simulink model "rx_20140505"  (R2012b)
settings: Solver=ode45  StartTime=0.0  StopTime=10000.0  RelTol=1e-3
libraries: xbsIndex_r4 x2064, casper_library_misc x67, xps_library x56, xbsReplacements_r4 x12, gavrt_library x3, casper_library_sources x2, simulink x1, casper_library_delays x1
(part 2 of 22)

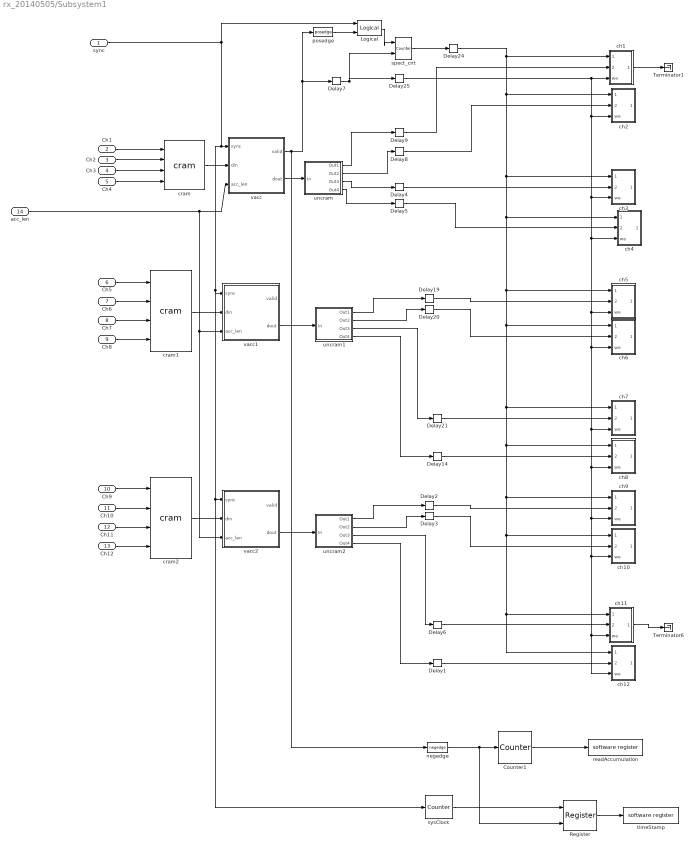
== system rx_20140505/Subsystem1 ==
  sync : Inport
  Ch1 : Inport  Port=2
  Ch2 : Inport  Port=3
  Ch3 : Inport  Port=4
  Ch4 : Inport  Port=5
  Ch5 : Inport  Port=6
  Ch6 : Inport  Port=7
  Ch7 : Inport  Port=8
  Ch8 : Inport  Port=9
  Ch9 : Inport  Port=10
  Ch10 : Inport  Port=11
  Ch11 : Inport  Port=12
  Ch12 : Inport  Port=13
  acc_len : Inport  Port=14
  Counter1 : xbsIndex_r4/Counter  cnt_type=Free Running  cnt_to=Inf  operation=Up  start_count=0  cnt_by_val=1  arith_type=Unsigned  n_bits=32  bin_pt=0  load_pin=off  rst=off  en=on  explicit_period=on  period=1  dbl_ovrd=off  use_behavioral_HDL=off  implementation=Fabric  block_type=counter
      settings: block_version=11.4
  Delay{1..6,8..9,14,19..21} (12 alike) : xbsIndex_r4/Delay  rst=off  infoeditControl=Selection of Reset will increase slice count due to use of real FFs and instead of SRLs  en=off  latency=2  dbl_ovrd=off  reg_retiming=on  block_type=delay
  Delay24 : xbsIndex_r4/Delay  rst=off  infoeditControl=Selection of Reset will increase slice count due to use of real FFs and instead of SRLs  en=off  latency=1  dbl_ovrd=off  reg_retiming=on  block_type=delay
  Delay25 : xbsIndex_r4/Delay  rst=off  infoeditControl=Selection of Reset will increase slice count due to use of real FFs and instead of SRLs  en=off  latency=1  dbl_ovrd=off  reg_retiming=on  block_type=delay
  Delay7 : xbsIndex_r4/Delay  rst=off  infoeditControl=Selection of Reset will increase slice count due to use of real FFs and instead of SRLs  en=off  latency=1  dbl_ovrd=off  reg_retiming=on  block_type=delay
  Logical : xbsIndex_r4/Logical  logical_function=OR  inputs=2  en=off  latency=0  precision=Full  arith_type=Unsigned  n_bits=16  bin_pt=0  align_bp=on  dbl_ovrd=off  block_type=logical
      settings: block_version=11.4
  Register : xbsIndex_r4/Register  init=0  rst=off  en=on  dbl_ovrd=off  block_type=register
      settings: block_version=11.4
  Terminator1 : Terminator
  Terminator6 : Terminator
  ch1 : Subsystem
  ch10 : Subsystem
  ch11 : Subsystem
  ch12 : Subsystem
  ch2 : Subsystem
  ch3 : Subsystem
  ch4 : Subsystem
  ch5 : Subsystem
  ch6 : Subsystem
  ch7 : Subsystem
  ch8 : Subsystem
  ch9 : Subsystem
  cram : gavrt_library/cram  num_slice=4
  cram1 : gavrt_library/cram  num_slice=4
  cram2 : gavrt_library/cram  num_slice=4
  negedge : casper_library_misc/negedge  Tag=Rising Edge Detector
  posedge : casper_library_misc/posedge  Tag=Rising Edge Detector
  readAccumulation : xps_library/software register  Tag=xps:sw_reg  io_dir=To Processor  arith_type=Unsigned  bitwidth=32  bin_pt=0  sample_period=1  gw_name=rx_20140505_Subsystem1_readAccumulation_user_data_in
  spect_cnt : xbsIndex_r4/Counter  cnt_type=Free Running  cnt_to=Inf  operation=Up  start_count=0  cnt_by_val=1  arith_type=Unsigned  n_bits=10  bin_pt=0  load_pin=off  rst=on  en=on  explicit_period=on  period=1  dbl_ovrd=off  use_behavioral_HDL=off  implementation=Fabric  use_rpm=off  block_type=counter
  sysClock : xbsIndex_r4/Counter  cnt_type=Free Running  cnt_to=Inf  operation=Up  start_count=0  cnt_by_val=1  arith_type=Unsigned  n_bits=32  bin_pt=0  load_pin=off  rst=on  en=off  explicit_period=on  period=1  dbl_ovrd=off  use_behavioral_HDL=off  implementation=Fabric  block_type=counter
      settings: block_version=11.4
  timeStamp : xps_library/software register  Tag=xps:sw_reg  io_dir=To Processor  arith_type=Unsigned  bitwidth=32  bin_pt=0  sample_period=1  gw_name=rx_20140505_Subsystem1_timeStamp_user_data_in
  uncram : Subsystem  AncestorBlock=gavrt_library/uncram  mask(uncram){num_slice=4, slice_width=64, bin_pt=0, arith_type=1}
      mask prompts: num_slice "Number of slices"; slice_width "Slice Width"; bin_pt "Output Binary Point"; arith_type "Output Arithmetic Type (0=Unsigned, 1=Signed)"
      mask help: Takes a concatenated input and slices it up into even pieces and reinterprets them as signed fixed point numbers with a given binary point.
      mask init:
      | uncram_init(gcb, ...
      |     'num_slice', num_slice, ...
      |     'slice_width', slice_width, ...
      |     'bin_pt', bin_pt, ...
      |     'arith_type', arith_type);
      settings: AttributesFormatString=Fix_64_0
  uncram1 : Subsystem  AncestorBlock=gavrt_library/uncram  mask(uncram){num_slice=4, slice_width=64, bin_pt=0, arith_type=1}
      mask prompts: num_slice "Number of slices"; slice_width "Slice Width"; bin_pt "Output Binary Point"; arith_type "Output Arithmetic Type (0=Unsigned, 1=Signed)"
      mask help: Takes a concatenated input and slices it up into even pieces and reinterprets them as signed fixed point numbers with a given binary point.
      mask init:
      | uncram_init(gcb, ...
      |     'num_slice', num_slice, ...
      |     'slice_width', slice_width, ...
      |     'bin_pt', bin_pt, ...
      |     'arith_type', arith_type);
      settings: AttributesFormatString=Fix_64_0
  uncram2 : Subsystem  AncestorBlock=gavrt_library/uncram  mask(uncram){num_slice=4, slice_width=64, bin_pt=0, arith_type=1}
      mask prompts: num_slice "Number of slices"; slice_width "Slice Width"; bin_pt "Output Binary Point"; arith_type "Output Arithmetic Type (0=Unsigned, 1=Signed)"
      mask help: Takes a concatenated input and slices it up into even pieces and reinterprets them as signed fixed point numbers with a given binary point.
      mask init:
      | uncram_init(gcb, ...
      |     'num_slice', num_slice, ...
      |     'slice_width', slice_width, ...
      |     'bin_pt', bin_pt, ...
      |     'arith_type', arith_type);
      settings: AttributesFormatString=Fix_64_0
  vacc : Subsystem  AncestorBlock=gavrt_library/vacc  mask(vacc){veclen=5, ninputs=4, max_accum=22, arith_type=1, in_bit_width=37, in_bin_pt=0, out_bit_width=64, out_bin_pt=0, register_din=0, add_latency=3, bram_latency=4, mux_latency=4}
      mask prompts: veclen "Vector Length (2^?)"; ninputs "Number of Simultaneous Vectors"; max_accum "Maximum # Accumulations (2^?)"; arith_type "Arithmetic Type (0=Unsigned, 1=Signed)"; in_bit_width "Input Bit Width"; in_bin_pt "Input Binary Point"; out_bit_width "Output Bit Width"; out_bin_pt "Output Binary Point"; register_din "Register Input Data  (1 = Enable Register Retiming on input delay)"; add_latency "Add Latency"; bram_latency "BRAM Latency"; mux_latency "Mux Latency"
      mask help:
      | Sync is expected the clock before the first data to be accumulated.
      | Use the Cram block to feed din for multiple simultaneous inputs.
      | acc_len is the number of vectors to sum.
      | valid is high while a valid accumulation is being clocked out on dout.
      | If only one sync pulse is provided, valid accumulations will repeatedly appear on dout as they become available.
      | Undesired behavior may occur if acc_len is changed without a new sync pulse.
      | Note: The output is an unsigned concatenation of the output streams. Thus, even with only one stream, the output must be recast before using.
      | Register Input Data controls the "Enable Register Retiming" parameter of the delays on 'din'.
      mask init:
      | vacc_init(gcb, ...
      |     'veclen', veclen, ...
      |     'ninputs', ninputs, ...
      |     'max_accum', max_accum, ...
      |     'arith_type', arith_type, ...
      |     'in_bit_width', in_bit_width, ...
      |     'in_bin_pt', in_bin_pt, ...
      |     'out_bit_width', out_bit_width, ...
      |     'out_bin_pt', out_bin_pt, ...
      |     'register_din', register_din, ...
      |     'add_latency', add_latency, ...
      |     'bram_latency', bram_latency, ...
      |     'mux_latency', mux_latency);
      settings: AttributesFormatString=|
      | vector length=32, inputs=4
      | max accumulations=2^22
  vacc1 : Subsystem  AncestorBlock=gavrt_library/vacc  mask(vacc){veclen=5, ninputs=4, max_accum=22, arith_type=1, in_bit_width=37, in_bin_pt=0, out_bit_width=64, out_bin_pt=0, register_din=0, add_latency=3, bram_latency=4, mux_latency=4}
      mask prompts: veclen "Vector Length (2^?)"; ninputs "Number of Simultaneous Vectors"; max_accum "Maximum # Accumulations (2^?)"; arith_type "Arithmetic Type (0=Unsigned, 1=Signed)"; in_bit_width "Input Bit Width"; in_bin_pt "Input Binary Point"; out_bit_width "Output Bit Width"; out_bin_pt "Output Binary Point"; register_din "Register Input Data  (1 = Enable Register Retiming on input delay)"; add_latency "Add Latency"; bram_latency "BRAM Latency"; mux_latency "Mux Latency"
      mask help:
      | Sync is expected the clock before the first data to be accumulated.
      | Use the Cram block to feed din for multiple simultaneous inputs.
      | acc_len is the number of vectors to sum.
      | valid is high while a valid accumulation is being clocked out on dout.
      | If only one sync pulse is provided, valid accumulations will repeatedly appear on dout as they become available.
      | Undesired behavior may occur if acc_len is changed without a new sync pulse.
      | Note: The output is an unsigned concatenation of the output streams. Thus, even with only one stream, the output must be recast before using.
      | Register Input Data controls the "Enable Register Retiming" parameter of the delays on 'din'.
      mask init: same as rx_20140505/Subsystem1/vacc
      settings: AttributesFormatString=|
      | vector length=32, inputs=4
      | max accumulations=2^22
  vacc2 : Subsystem  AncestorBlock=gavrt_library/vacc  mask(vacc){veclen=5, ninputs=4, max_accum=22, arith_type=1, in_bit_width=37, in_bin_pt=0, out_bit_width=64, out_bin_pt=0, register_din=0, add_latency=3, bram_latency=4, mux_latency=4}
      mask prompts: veclen "Vector Length (2^?)"; ninputs "Number of Simultaneous Vectors"; max_accum "Maximum # Accumulations (2^?)"; arith_type "Arithmetic Type (0=Unsigned, 1=Signed)"; in_bit_width "Input Bit Width"; in_bin_pt "Input Binary Point"; out_bit_width "Output Bit Width"; out_bin_pt "Output Binary Point"; register_din "Register Input Data  (1 = Enable Register Retiming on input delay)"; add_latency "Add Latency"; bram_latency "BRAM Latency"; mux_latency "Mux Latency"
      mask help:
      | Sync is expected the clock before the first data to be accumulated.
      | Use the Cram block to feed din for multiple simultaneous inputs.
      | acc_len is the number of vectors to sum.
      | valid is high while a valid accumulation is being clocked out on dout.
      | If only one sync pulse is provided, valid accumulations will repeatedly appear on dout as they become available.
      | Undesired behavior may occur if acc_len is changed without a new sync pulse.
      | Note: The output is an unsigned concatenation of the output streams. Thus, even with only one stream, the output must be recast before using.
      | Register Input Data controls the "Enable Register Retiming" parameter of the delays on 'din'.
      mask init: same as rx_20140505/Subsystem1/vacc
      settings: AttributesFormatString=|
      | vector length=32, inputs=4
      | max accumulations=2^22
  wires:
  ch1/1(Out1) -> Terminator1/1
  Delay4/1 -> ch3/2(data)
  uncram1/2(Out2) -> Delay20/1
  uncram1/3(Out3) -> Delay21/1
  Ch3/1 -> cram/3
  Ch4/1 -> cram/4
  Ch2/1 -> cram/2
  Ch1/1 -> cram/1
  cram/1 -> vacc/2(din)
  vacc/1(valid) -> posedge/1, Delay7/1, negedge/1
  Delay7/1 -> spect_cnt/2, Delay25/1
  vacc/2(dout) -> uncram/1(In)
  uncram/1(Out1) -> Delay9/1
  uncram/2(Out2) -> Delay8/1
  uncram/3(Out3) -> Delay4/1
  uncram/4(Out4) -> Delay5/1
  Delay8/1 -> ch2/2(data)
  Delay9/1 -> ch1/2(data)
  spect_cnt/1 -> Delay24/1
  Delay24/1 -> ch1/1(addr), ch2/1(addr), ch3/1(addr), ch4/1(addr), ch5/1(addr), ch6/1(addr), ch7/1(addr), ch8/1(addr), ch9/1(addr), ch10/1(addr), ch12/1(addr), ch11/1(addr)
  Delay25/1 -> ch1/3(we), ch2/3(we), ch3/3(we), ch4/3(we), ch5/3(we), ch6/3(we), ch7/3(we), ch8/3(we), ch9/3(we), ch10/3(we), ch12/3(we), ch11/3(we)
  Delay5/1 -> ch4/2(data)
  Ch5/1 -> cram1/1
  Ch6/1 -> cram1/2
  Ch7/1 -> cram1/3
  Ch8/1 -> cram1/4
  cram1/1 -> vacc1/2(din)
  vacc1/2(dout) -> uncram1/1(In)
  uncram1/1(Out1) -> Delay19/1
  uncram1/4(Out4) -> Delay14/1
  Delay19/1 -> ch5/2(data)
  Delay20/1 -> ch6/2(data)
  Delay21/1 -> ch7/2(data)
  Delay14/1 -> ch8/2(data)
  sync/1 -> vacc/1(sync), vacc1/1(sync), vacc2/1(sync), sysClock/1, Logical/1
  acc_len/1 -> vacc/3(acc_len), vacc2/3(acc_len), vacc1/3(acc_len)
  negedge/1 -> Counter1/1, Register/2
  Counter1/1 -> readAccumulation/1
  uncram2/2(Out2) -> Delay3/1
  uncram2/3(Out3) -> Delay6/1
  ch11/1(Out1) -> Terminator6/1
  Ch9/1 -> cram2/1
  Ch10/1 -> cram2/2
  Ch11/1 -> cram2/3
  Ch12/1 -> cram2/4
  cram2/1 -> vacc2/2(din)
  vacc2/2(dout) -> uncram2/1(In)
  uncram2/1(Out1) -> Delay2/1
  uncram2/4(Out4) -> Delay1/1
  Delay2/1 -> ch9/2(data)
  Delay3/1 -> ch10/2(data)
  Delay6/1 -> ch11/2(data)
  Delay1/1 -> ch12/2(data)
  Register/1 -> timeStamp/1
  sysClock/1 -> Register/1
  posedge/1 -> Logical/2
  Logical/1 -> spect_cnt/1

== system rx_20140505/Subsystem2 ==
  In1 : Inport
  In2 : Inport  Port=2
  AddSub : xbsIndex_r4/AddSub  mode=Addition  use_carryin=off  use_carryout=off  en=off  latency=2  precision=Full  arith_type=Unsigned  n_bits=16  bin_pt=14  quantization=Truncate  overflow=Wrap  dbl_ovrd=off  use_behavioral_HDL=off  hw_selection=Fabric  pipelined=off  block_type=addsub
  AddSub1 : xbsIndex_r4/AddSub  mode=Addition  use_carryin=off  use_carryout=off  en=off  latency=2  precision=Full  arith_type=Unsigned  n_bits=16  bin_pt=14  quantization=Truncate  overflow=Wrap  dbl_ovrd=off  use_behavioral_HDL=off  hw_selection=Fabric  pipelined=off  block_type=addsub
  AddSub2 : xbsIndex_r4/AddSub  mode=Subtraction  use_carryin=off  use_carryout=off  en=off  latency=2  precision=Full  arith_type=Unsigned  n_bits=16  bin_pt=14  quantization=Truncate  overflow=Wrap  dbl_ovrd=off  use_behavioral_HDL=off  hw_selection=Fabric  pipelined=off  block_type=addsub
  AddSub3 : xbsIndex_r4/AddSub  mode=Subtraction  use_carryin=off  use_carryout=off  en=off  latency=2  precision=Full  arith_type=Unsigned  n_bits=16  bin_pt=14  quantization=Truncate  overflow=Wrap  dbl_ovrd=off  use_behavioral_HDL=off  hw_selection=Fabric  pipelined=off  block_type=addsub
  Slice{,1..2,21} (4 alike) : xbsIndex_r4/Slice  nbits=18  boolean_output=off  mode=Upper Bit Location + Width  bit1=0  base1=MSB of Input  bit0=0  base0=LSB of Input  dbl_ovrd=off  block_type=slice
  c_to_ri1 : casper_library_misc/c_to_ri  n_bits=18  bin_pt=0
      settings: AttributesFormatString=18_0 r/i
  c_to_ri2 : casper_library_misc/c_to_ri  n_bits=18  bin_pt=0
      settings: AttributesFormatString=18_0 r/i
  ri_to_c : casper_library_misc/ri_to_c
  ri_to_c1 : casper_library_misc/ri_to_c
  Add : Outport
  Subtract : Outport  Port=2
  wires:
  c_to_ri1/1 -> AddSub/1, AddSub2/1
  c_to_ri2/1 -> AddSub/2, AddSub2/2
  c_to_ri1/2 -> AddSub1/1, AddSub3/1
  c_to_ri2/2 -> AddSub1/2, AddSub3/2
  Slice/1 -> ri_to_c/1
  AddSub/1 -> Slice/1
  AddSub1/1 -> Slice21/1
  In1/1 -> c_to_ri1/1
  ri_to_c/1 -> Add/1
  Slice21/1 -> ri_to_c/2
  In2/1 -> c_to_ri2/1
  Slice1/1 -> ri_to_c1/1
  AddSub2/1 -> Slice1/1
  AddSub3/1 -> Slice2/1
  Slice2/1 -> ri_to_c1/2
  ri_to_c1/1 -> Subtract/1

== system rx_20140505/Subsystem3 ==
  In1 : Inport
  In2 : Inport  Port=2
  AddSub : xbsIndex_r4/AddSub  mode=Addition  use_carryin=off  use_carryout=off  en=off  latency=2  precision=Full  arith_type=Unsigned  n_bits=16  bin_pt=14  quantization=Truncate  overflow=Wrap  dbl_ovrd=off  use_behavioral_HDL=off  hw_selection=Fabric  pipelined=off  block_type=addsub
  AddSub1 : xbsIndex_r4/AddSub  mode=Addition  use_carryin=off  use_carryout=off  en=off  latency=2  precision=Full  arith_type=Unsigned  n_bits=16  bin_pt=14  quantization=Truncate  overflow=Wrap  dbl_ovrd=off  use_behavioral_HDL=off  hw_selection=Fabric  pipelined=off  block_type=addsub
  AddSub2 : xbsIndex_r4/AddSub  mode=Subtraction  use_carryin=off  use_carryout=off  en=off  latency=2  precision=Full  arith_type=Unsigned  n_bits=16  bin_pt=14  quantization=Truncate  overflow=Wrap  dbl_ovrd=off  use_behavioral_HDL=off  hw_selection=Fabric  pipelined=off  block_type=addsub
  AddSub3 : xbsIndex_r4/AddSub  mode=Subtraction  use_carryin=off  use_carryout=off  en=off  latency=2  precision=Full  arith_type=Unsigned  n_bits=16  bin_pt=14  quantization=Truncate  overflow=Wrap  dbl_ovrd=off  use_behavioral_HDL=off  hw_selection=Fabric  pipelined=off  block_type=addsub
  Slice{,1..2,21} (4 alike) : xbsIndex_r4/Slice  nbits=18  boolean_output=off  mode=Upper Bit Location + Width  bit1=0  base1=MSB of Input  bit0=0  base0=LSB of Input  dbl_ovrd=off  block_type=slice
  c_to_ri1 : casper_library_misc/c_to_ri  n_bits=18  bin_pt=0
      settings: AttributesFormatString=18_0 r/i
  c_to_ri2 : casper_library_misc/c_to_ri  n_bits=18  bin_pt=0
      settings: AttributesFormatString=18_0 r/i
  ri_to_c : casper_library_misc/ri_to_c
  ri_to_c1 : casper_library_misc/ri_to_c
  Add : Outport
  Subtract : Outport  Port=2
  wires:
  c_to_ri1/1 -> AddSub/1, AddSub2/1
  c_to_ri2/1 -> AddSub/2, AddSub2/2
  c_to_ri1/2 -> AddSub1/1, AddSub3/1
  c_to_ri2/2 -> AddSub1/2, AddSub3/2
  Slice/1 -> ri_to_c/1
  AddSub/1 -> Slice/1
  AddSub1/1 -> Slice21/1
  In1/1 -> c_to_ri1/1
  ri_to_c/1 -> Add/1
  Slice21/1 -> ri_to_c/2
  In2/1 -> c_to_ri2/1
  Slice1/1 -> ri_to_c1/1
  AddSub2/1 -> Slice1/1
  AddSub3/1 -> Slice2/1
  Slice2/1 -> ri_to_c1/2
  ri_to_c1/1 -> Subtract/1

== system rx_20140505/Subsystem4 ==
  In1 : Inport
  In2 : Inport  Port=2
  AddSub : xbsIndex_r4/AddSub  mode=Addition  use_carryin=off  use_carryout=off  en=off  latency=2  precision=Full  arith_type=Unsigned  n_bits=16  bin_pt=14  quantization=Truncate  overflow=Wrap  dbl_ovrd=off  use_behavioral_HDL=off  hw_selection=Fabric  pipelined=off  block_type=addsub
  AddSub1 : xbsIndex_r4/AddSub  mode=Addition  use_carryin=off  use_carryout=off  en=off  latency=2  precision=Full  arith_type=Unsigned  n_bits=16  bin_pt=14  quantization=Truncate  overflow=Wrap  dbl_ovrd=off  use_behavioral_HDL=off  hw_selection=Fabric  pipelined=off  block_type=addsub
  AddSub2 : xbsIndex_r4/AddSub  mode=Subtraction  use_carryin=off  use_carryout=off  en=off  latency=2  precision=Full  arith_type=Unsigned  n_bits=16  bin_pt=14  quantization=Truncate  overflow=Wrap  dbl_ovrd=off  use_behavioral_HDL=off  hw_selection=Fabric  pipelined=off  block_type=addsub
  AddSub3 : xbsIndex_r4/AddSub  mode=Subtraction  use_carryin=off  use_carryout=off  en=off  latency=2  precision=Full  arith_type=Unsigned  n_bits=16  bin_pt=14  quantization=Truncate  overflow=Wrap  dbl_ovrd=off  use_behavioral_HDL=off  hw_selection=Fabric  pipelined=off  block_type=addsub
  Slice{,1..2,21} (4 alike) : xbsIndex_r4/Slice  nbits=18  boolean_output=off  mode=Upper Bit Location + Width  bit1=0  base1=MSB of Input  bit0=0  base0=LSB of Input  dbl_ovrd=off  block_type=slice
  c_to_ri1 : casper_library_misc/c_to_ri  n_bits=18  bin_pt=0
      settings: AttributesFormatString=18_0 r/i
  c_to_ri2 : casper_library_misc/c_to_ri  n_bits=18  bin_pt=0
      settings: AttributesFormatString=18_0 r/i
  ri_to_c : casper_library_misc/ri_to_c
  ri_to_c1 : casper_library_misc/ri_to_c
  Add : Outport
  Subtract : Outport  Port=2
  wires:
  c_to_ri1/1 -> AddSub/1, AddSub2/1
  c_to_ri2/1 -> AddSub/2, AddSub2/2
  c_to_ri1/2 -> AddSub1/1, AddSub3/1
  c_to_ri2/2 -> AddSub1/2, AddSub3/2
  Slice/1 -> ri_to_c/1
  AddSub/1 -> Slice/1
  AddSub1/1 -> Slice21/1
  In1/1 -> c_to_ri1/1
  ri_to_c/1 -> Add/1
  Slice21/1 -> ri_to_c/2
  In2/1 -> c_to_ri2/1
  Slice1/1 -> ri_to_c1/1
  AddSub2/1 -> Slice1/1
  AddSub3/1 -> Slice2/1
  Slice2/1 -> ri_to_c1/2
  ri_to_c1/1 -> Subtract/1

== system rx_20140505/Subsystem5 ==
  In1 : Inport
  In2 : Inport  Port=2
  AddSub : xbsIndex_r4/AddSub  mode=Addition  use_carryin=off  use_carryout=off  en=off  latency=2  precision=Full  arith_type=Unsigned  n_bits=16  bin_pt=14  quantization=Truncate  overflow=Wrap  dbl_ovrd=off  use_behavioral_HDL=off  hw_selection=Fabric  pipelined=off  block_type=addsub
  AddSub1 : xbsIndex_r4/AddSub  mode=Addition  use_carryin=off  use_carryout=off  en=off  latency=2  precision=Full  arith_type=Unsigned  n_bits=16  bin_pt=14  quantization=Truncate  overflow=Wrap  dbl_ovrd=off  use_behavioral_HDL=off  hw_selection=Fabric  pipelined=off  block_type=addsub
  AddSub2 : xbsIndex_r4/AddSub  mode=Subtraction  use_carryin=off  use_carryout=off  en=off  latency=2  precision=Full  arith_type=Unsigned  n_bits=16  bin_pt=14  quantization=Truncate  overflow=Wrap  dbl_ovrd=off  use_behavioral_HDL=off  hw_selection=Fabric  pipelined=off  block_type=addsub
  AddSub3 : xbsIndex_r4/AddSub  mode=Subtraction  use_carryin=off  use_carryout=off  en=off  latency=2  precision=Full  arith_type=Unsigned  n_bits=16  bin_pt=14  quantization=Truncate  overflow=Wrap  dbl_ovrd=off  use_behavioral_HDL=off  hw_selection=Fabric  pipelined=off  block_type=addsub
  Slice{,1..2,21} (4 alike) : xbsIndex_r4/Slice  nbits=18  boolean_output=off  mode=Upper Bit Location + Width  bit1=0  base1=MSB of Input  bit0=0  base0=LSB of Input  dbl_ovrd=off  block_type=slice
  c_to_ri1 : casper_library_misc/c_to_ri  n_bits=18  bin_pt=0
      settings: AttributesFormatString=18_0 r/i
  c_to_ri2 : casper_library_misc/c_to_ri  n_bits=18  bin_pt=0
      settings: AttributesFormatString=18_0 r/i
  ri_to_c : casper_library_misc/ri_to_c
  ri_to_c1 : casper_library_misc/ri_to_c
  Add : Outport
  Subtract : Outport  Port=2
  wires:
  c_to_ri1/1 -> AddSub/1, AddSub2/1
  c_to_ri2/1 -> AddSub/2, AddSub2/2
  c_to_ri1/2 -> AddSub1/1, AddSub3/1
  c_to_ri2/2 -> AddSub1/2, AddSub3/2
  Slice/1 -> ri_to_c/1
  AddSub/1 -> Slice/1
  AddSub1/1 -> Slice21/1
  In1/1 -> c_to_ri1/1
  ri_to_c/1 -> Add/1
  Slice21/1 -> ri_to_c/2
  In2/1 -> c_to_ri2/1
  Slice1/1 -> ri_to_c1/1
  AddSub2/1 -> Slice1/1
  AddSub3/1 -> Slice2/1
  Slice2/1 -> ri_to_c1/2
  ri_to_c1/1 -> Subtract/1

== system rx_20140505/Walshing1 ==
  CLK : Inport
  Delay9 : xbsIndex_r4/Delay  rst=off  infoeditControl=Selection of Reset will increase slice count due to use of real FFs and instead of SRLs  en=off  latency=1  dbl_ovrd=off  reg_retiming=off  block_type=delay
  Inverter : xbsIndex_r4/Inverter  en=off  latency=0  dbl_ovrd=off  block_type=inv
      settings: block_version=11.4
  Inverter1 : xbsIndex_r4/Inverter  en=off  latency=0  dbl_ovrd=off  block_type=inv
      settings: block_version=11.4
  Inverter2 : xbsIndex_r4/Inverter  en=off  latency=0  dbl_ovrd=off  block_type=inv
      settings: block_version=11.4
  JK FlipFlop2 : Subsystem
  Logical{1..4} (4 alike) : xbsIndex_r4/Logical  logical_function=XOR  inputs=2  en=off  latency=0  precision=Full  arith_type=Unsigned  n_bits=16  bin_pt=0  align_bp=on  dbl_ovrd=off  block_type=logical
      settings: block_version=11.4
  Scope4 : Scope  NumInputPorts=7
      settings: YMin=0~-5~-5~-5~-5~-5~-5  YMax=1~5~5~5~5~5~5  SaveName=ScopeData5
  out : xbsIndex_r4/Gateway Out  inherit_from_input=off  hdl_port=on  timing_constraint=None  locs_specified=off  LOCs={}  UseAsDAC=off  DACChannel='1'  block_type=gatewayout
      settings: infoedit="Gateway out block.  Converts Xilinx fixed point inputs into ouputs of type Simulink integer, double, or fixed point.<br><br>Hardware notes:  In hardware these blocks become top level output ports or are discarded, depending on how they are configured."  block_version=11.4
  out1 : xbsIndex_r4/Gateway Out  inherit_from_input=off  hdl_port=on  timing_constraint=None  locs_specified=off  LOCs={}  UseAsDAC=off  DACChannel='1'  block_type=gatewayout
      settings: infoedit="Gateway out block.  Converts Xilinx fixed point inputs into ouputs of type Simulink integer, double, or fixed point.<br><br>Hardware notes:  In hardware these blocks become top level output ports or are discarded, depending on how they are configured."  block_version=11.4
  out2 : xbsIndex_r4/Gateway Out  inherit_from_input=off  hdl_port=on  timing_constraint=None  locs_specified=off  LOCs={}  UseAsDAC=off  DACChannel='1'  block_type=gatewayout
      settings: infoedit="Gateway out block.  Converts Xilinx fixed point inputs into ouputs of type Simulink integer, double, or fixed point.<br><br>Hardware notes:  In hardware these blocks become top level output ports or are discarded, depending on how they are configured."  block_version=11.4
  Out1 : Outport
  Out2 : Outport  Port=2
  Out3 : Outport  Port=3
  Out4 : Outport  Port=4
  Out5 : Outport  Port=5
  Out6 : Outport  Port=6
  Out7 : Outport  Port=7
  wires:
  JK FlipFlop2/2(CLK/4) -> Logical2/1, Out1/1, Logical4/1, out2/1
  CLK/1 -> JK FlipFlop2/1(CLK), Delay9/1
  JK FlipFlop2/1(CLK/2) -> Logical2/2, Out3/1, Logical1/1, out1/1
  Logical2/1 -> Inverter/1, Logical3/1
  Inverter/1 -> Out2/1
  Logical1/1 -> Inverter1/1
  Inverter1/1 -> Out4/1
  Logical3/1 -> Out5/1
  Logical4/1 -> Inverter2/1
  Inverter2/1 -> Out6/1
  Delay9/1 -> Logical1/2, Logical3/2, Logical4/2, Out7/1, out/1
  out/1 -> Scope4/1
  out1/1 -> Scope4/2
  out2/1 -> Scope4/3

== system rx_20140505/amp_EQ0 ==
  sync_in : Inport
  din : Inport  Port=2
  Concat : xbsIndex_r4/Concat  num_inputs=2  dbl_ovrd=off  block_type=concat
  Concat1 : xbsIndex_r4/Concat  num_inputs=2  dbl_ovrd=off  block_type=concat
  Constant : xbsIndex_r4/Constant  const=0  gui_display_data_type=Fixed-point  arith_type=Boolean  n_bits=16  bin_pt=14  preci_type=Single  exp_width=8  frac_width=24  explicit_period=on  period=1  equ=P=C  opselect=C  inp2=PCIN>>17  opr=+  inp1=P  carry=CIN  dbl_ovrd=off  block_type=constant
      settings: block_version=11.4
  Constant1 : xbsIndex_r4/Constant  const=0  gui_display_data_type=Fixed-point  arith_type=Unsigned  n_bits=32  bin_pt=0  preci_type=Single  exp_width=8  frac_width=24  explicit_period=on  period=1  equ=P=C  opselect=C  inp2=PCIN>>17  opr=+  inp1=P  carry=CIN  dbl_ovrd=off  block_type=constant
      settings: block_version=11.4
  Constant2 : xbsIndex_r4/Constant  const=0  gui_display_data_type=Fixed-point  arith_type=Boolean  n_bits=16  bin_pt=14  preci_type=Single  exp_width=8  frac_width=24  explicit_period=on  period=1  equ=P=C  opselect=C  inp2=PCIN>>17  opr=+  inp1=P  carry=CIN  dbl_ovrd=off  block_type=constant
      settings: block_version=11.4
  Constant3 : xbsIndex_r4/Constant  const=0  gui_display_data_type=Fixed-point  arith_type=Unsigned  n_bits=32  bin_pt=0  preci_type=Single  exp_width=8  frac_width=24  explicit_period=on  period=1  equ=P=C  opselect=C  inp2=PCIN>>17  opr=+  inp1=P  carry=CIN  dbl_ovrd=off  block_type=constant
      settings: block_version=11.4
  Counter : xbsIndex_r4/Counter  cnt_type=Free Running  cnt_to=Inf  operation=Up  start_count=0  cnt_by_val=1  arith_type=Unsigned  n_bits=N  bin_pt=0  load_pin=off  rst=on  en=off  explicit_period=on  period=1  dbl_ovrd=off  use_behavioral_HDL=off  implementation=Fabric  block_type=counter
      settings: block_version=11.4
  Delay1 : xbsIndex_r4/Delay  rst=off  infoeditControl=Selection of Reset will increase slice count due to use of real FFs and instead of SRLs  en=off  latency=1  dbl_ovrd=off  reg_retiming=off  block_type=delay
      settings: block_version=11.4
  Delay2 : xbsIndex_r4/Delay  rst=off  infoeditControl=Selection of Reset will increase slice count due to use of real FFs and instead of SRLs  en=off  latency=1  dbl_ovrd=off  reg_retiming=off  block_type=delay
      settings: block_version=11.4
  Reinterpret : xbsIndex_r4/Reinterpret  force_arith_type=on  arith_type="Signed  (2's comp)"  force_bin_pt=off  bin_pt=0  block_type=reinterpret
      settings: infoedit="Changes signal type without altering the binary representation.   You can changed the signal between signed and unsigned, and relocate the binary point.<br><br>Hardware notes: In hardware this block costs nothing.<br><br>Example:  Suppose the input is 6 bits wide, signed, with 2 fractional bits, and the output is forced to unsigned with 0 fractional bits.  Then an input of -2.0 (1110.00 in binary 2's complement) becomes an output of 56 (111000 in binary)."
  Reinterpret1 : xbsIndex_r4/Reinterpret  force_arith_type=on  arith_type="Signed  (2's comp)"  force_bin_pt=off  bin_pt=0  block_type=reinterpret
      settings: infoedit="Changes signal type without altering the binary representation.   You can changed the signal between signed and unsigned, and relocate the binary point.<br><br>Hardware notes: In hardware this block costs nothing.<br><br>Example:  Suppose the input is 6 bits wide, signed, with 2 fractional bits, and the output is forced to unsigned with 0 fractional bits.  Then an input of -2.0 (1110.00 in binary 2's complement) becomes an output of 56 (111000 in binary)."
  Slice : xbsIndex_r4/Slice  nbits=1  boolean_output=off  mode=Upper Bit Location + Width  bit1=0  base1=MSB of Input  bit0=0  base0=LSB of Input  dbl_ovrd=off  block_type=slice
  Slice1 : xbsIndex_r4/Slice  nbits=1  boolean_output=off  mode=Upper Bit Location + Width  bit1=0  base1=MSB of Input  bit0=0  base0=LSB of Input  dbl_ovrd=off  block_type=slice
  Slice2 : xbsIndex_r4/Slice  nbits=12  boolean_output=off  mode=Lower Bit Location + Width  bit1=0  base1=MSB of Input  bit0=0  base0=LSB of Input  dbl_ovrd=off  block_type=slice
  Slice3 : xbsIndex_r4/Slice  nbits=12  boolean_output=off  mode=Lower Bit Location + Width  bit1=0  base1=MSB of Input  bit0=0  base0=LSB of Input  dbl_ovrd=off  block_type=slice
  amp_scale : Subsystem  mask{add_latency=2, mult_latency=3, bit_width=18, scale_bit_width=13}
      mask prompts: bit_width "bit_width_data"; scale_bit_width "bit_width_Scaling"
      mask init:
      | add_latency=2;
      | mult_latency=3;
  coeff_imag : Subsystem  Tag=xps:bram  AncestorBlock=xps_library/Shared BRAM  mask{arith_type=Unsigned, addr_width=10, data_width=32, reg_prim_output=on, reg_core_output=on, optimization=Minimum_Area, data_bin_pt=0, init_vals=[0:2^10-1], sample_rate=1}
      mask prompts: arith_type "Output Data Type"; addr_width "Address width"; data_width "Data Width"; reg_prim_output "Register Primitive Output"; reg_core_output "Register Core Output"; data_bin_pt "Data Binary Point"; init_vals "Initial 32-bit values (simulation only)"; sample_rate "Sample rate"
      mask init:
      | shared_bram_mask;
      mask TypeOptions arith_type: Unsigned | Signed  (2's comp)
      mask TypeOptions data_width: 8 | 16 | 32 | 64 | 128
      mask TypeOptions optimization: Minimum_Area | Low_Power
  coeff_real : Subsystem  Tag=xps:bram  AncestorBlock=xps_library/Shared BRAM  mask{arith_type=Unsigned, addr_width=10, data_width=32, reg_prim_output=on, reg_core_output=on, optimization=Minimum_Area, data_bin_pt=0, init_vals=[0:2^10-1], sample_rate=1}
      mask prompts: arith_type "Output Data Type"; addr_width "Address width"; data_width "Data Width"; reg_prim_output "Register Primitive Output"; reg_core_output "Register Core Output"; data_bin_pt "Data Binary Point"; init_vals "Initial 32-bit values (simulation only)"; sample_rate "Sample rate"
      mask init:
      | shared_bram_mask;
      mask TypeOptions arith_type: Unsigned | Signed  (2's comp)
      mask TypeOptions data_width: 8 | 16 | 32 | 64 | 128
      mask TypeOptions optimization: Minimum_Area | Low_Power
  pipeline1 : Subsystem  AncestorBlock=casper_library_delays/pipeline  mask(pipeline){latency=1}
      mask help:
      | An explicitly laid-out delay line to avoid mapping to SRL16s
      | for use in pipelining to help achieve timing closure.
      mask init:
      | pipeline_init(gcb,'latency',latency);
      settings: AttributesFormatString=Latency = %<latency>
      mask Display:
      | port_label('input', 1, 'd');
      | port_label('output', 1, 'q');
      | disp(['Z^-', num2str(latency)]);
  pipeline2 : Subsystem  AncestorBlock=casper_library_delays/pipeline  mask(pipeline){latency=1}
      mask help:
      | An explicitly laid-out delay line to avoid mapping to SRL16s
      | for use in pipelining to help achieve timing closure.
      mask init:
      | pipeline_init(gcb,'latency',latency);
      settings: AttributesFormatString=Latency = %<latency>
      mask Display:
      | port_label('input', 1, 'd');
      | port_label('output', 1, 'q');
      | disp(['Z^-', num2str(latency)]);
  ri_to_c : casper_library_misc/ri_to_c
  dout : Outport
  sync_out : Outport  Port=2
  wires:
  Counter/1 -> coeff_imag/1(addr), coeff_real/1(addr)
  sync_in/1 -> Counter/1, amp_scale/1(sync)
  Constant/1 -> coeff_real/3(we)
  Constant1/1 -> coeff_real/2(data_in)
  Constant3/1 -> coeff_imag/2(data_in)
  Constant2/1 -> coeff_imag/3(we)
  din/1 -> Delay1/1
  amp_scale/2(Out) -> dout/1
  ri_to_c/1 -> amp_scale/3(scale)
  amp_scale/1(synchOut) -> sync_out/1
  Delay1/1 -> Delay2/1
  Delay2/1 -> amp_scale/2(din)
  Slice/1 -> Concat/1
  Slice3/1 -> Concat/2
  Concat/1 -> Reinterpret/1
  pipeline2/1(q) -> Slice3/1, Slice/1
  Slice1/1 -> Concat1/1
  Slice2/1 -> Concat1/2
  Concat1/1 -> Reinterpret1/1
  pipeline1/1(q) -> Slice1/1, Slice2/1
  coeff_real/1(data_out) -> pipeline2/1(d)
  coeff_imag/1(data_out) -> pipeline1/1(d)
  Reinterpret/1 -> ri_to_c/1
  Reinterpret1/1 -> ri_to_c/2

== system rx_20140505/amp_EQ1 ==
  sync_in : Inport
  din : Inport  Port=2
  Concat : xbsIndex_r4/Concat  num_inputs=2  dbl_ovrd=off  block_type=concat
  Concat1 : xbsIndex_r4/Concat  num_inputs=2  dbl_ovrd=off  block_type=concat
  Constant : xbsIndex_r4/Constant  const=0  gui_display_data_type=Fixed-point  arith_type=Boolean  n_bits=16  bin_pt=14  preci_type=Single  exp_width=8  frac_width=24  explicit_period=on  period=1  equ=P=C  opselect=C  inp2=PCIN>>17  opr=+  inp1=P  carry=CIN  dbl_ovrd=off  block_type=constant
      settings: block_version=11.4
  Constant1 : xbsIndex_r4/Constant  const=0  gui_display_data_type=Fixed-point  arith_type=Unsigned  n_bits=32  bin_pt=0  preci_type=Single  exp_width=8  frac_width=24  explicit_period=on  period=1  equ=P=C  opselect=C  inp2=PCIN>>17  opr=+  inp1=P  carry=CIN  dbl_ovrd=off  block_type=constant
      settings: block_version=11.4
  Constant2 : xbsIndex_r4/Constant  const=0  gui_display_data_type=Fixed-point  arith_type=Boolean  n_bits=16  bin_pt=14  preci_type=Single  exp_width=8  frac_width=24  explicit_period=on  period=1  equ=P=C  opselect=C  inp2=PCIN>>17  opr=+  inp1=P  carry=CIN  dbl_ovrd=off  block_type=constant
      settings: block_version=11.4
  Constant3 : xbsIndex_r4/Constant  const=0  gui_display_data_type=Fixed-point  arith_type=Unsigned  n_bits=32  bin_pt=0  preci_type=Single  exp_width=8  frac_width=24  explicit_period=on  period=1  equ=P=C  opselect=C  inp2=PCIN>>17  opr=+  inp1=P  carry=CIN  dbl_ovrd=off  block_type=constant
      settings: block_version=11.4
  Counter : xbsIndex_r4/Counter  cnt_type=Free Running  cnt_to=Inf  operation=Up  start_count=0  cnt_by_val=1  arith_type=Unsigned  n_bits=N  bin_pt=0  load_pin=off  rst=on  en=off  explicit_period=on  period=1  dbl_ovrd=off  use_behavioral_HDL=off  implementation=Fabric  block_type=counter
      settings: block_version=11.4
  Delay1 : xbsIndex_r4/Delay  rst=off  infoeditControl=Selection of Reset will increase slice count due to use of real FFs and instead of SRLs  en=off  latency=1  dbl_ovrd=off  reg_retiming=off  block_type=delay
      settings: block_version=11.4
  Delay2 : xbsIndex_r4/Delay  rst=off  infoeditControl=Selection of Reset will increase slice count due to use of real FFs and instead of SRLs  en=off  latency=1  dbl_ovrd=off  reg_retiming=off  block_type=delay
      settings: block_version=11.4
  Reinterpret : xbsIndex_r4/Reinterpret  force_arith_type=on  arith_type="Signed  (2's comp)"  force_bin_pt=off  bin_pt=0  block_type=reinterpret
      settings: infoedit="Changes signal type without altering the binary representation.   You can changed the signal between signed and unsigned, and relocate the binary point.<br><br>Hardware notes: In hardware this block costs nothing.<br><br>Example:  Suppose the input is 6 bits wide, signed, with 2 fractional bits, and the output is forced to unsigned with 0 fractional bits.  Then an input of -2.0 (1110.00 in binary 2's complement) becomes an output of 56 (111000 in binary)."
  Reinterpret1 : xbsIndex_r4/Reinterpret  force_arith_type=on  arith_type="Signed  (2's comp)"  force_bin_pt=off  bin_pt=0  block_type=reinterpret
      settings: infoedit="Changes signal type without altering the binary representation.   You can changed the signal between signed and unsigned, and relocate the binary point.<br><br>Hardware notes: In hardware this block costs nothing.<br><br>Example:  Suppose the input is 6 bits wide, signed, with 2 fractional bits, and the output is forced to unsigned with 0 fractional bits.  Then an input of -2.0 (1110.00 in binary 2's complement) becomes an output of 56 (111000 in binary)."
  Slice : xbsIndex_r4/Slice  nbits=1  boolean_output=off  mode=Upper Bit Location + Width  bit1=0  base1=MSB of Input  bit0=0  base0=LSB of Input  dbl_ovrd=off  block_type=slice
  Slice1 : xbsIndex_r4/Slice  nbits=1  boolean_output=off  mode=Upper Bit Location + Width  bit1=0  base1=MSB of Input  bit0=0  base0=LSB of Input  dbl_ovrd=off  block_type=slice
  Slice2 : xbsIndex_r4/Slice  nbits=12  boolean_output=off  mode=Lower Bit Location + Width  bit1=0  base1=MSB of Input  bit0=0  base0=LSB of Input  dbl_ovrd=off  block_type=slice
  Slice3 : xbsIndex_r4/Slice  nbits=12  boolean_output=off  mode=Lower Bit Location + Width  bit1=0  base1=MSB of Input  bit0=0  base0=LSB of Input  dbl_ovrd=off  block_type=slice
  amp_scale : Subsystem  mask{add_latency=2, mult_latency=3, bit_width=18, scale_bit_width=13}
      mask prompts: bit_width "bit_width_data"; scale_bit_width "bit_width_Scaling"
      mask init:
      | add_latency=2;
      | mult_latency=3;
  coeff_imag : Subsystem  Tag=xps:bram  AncestorBlock=xps_library/Shared BRAM  mask{arith_type=Unsigned, addr_width=10, data_width=32, reg_prim_output=on, reg_core_output=on, optimization=Minimum_Area, data_bin_pt=0, init_vals=[0:2^10-1], sample_rate=1}
      mask prompts: arith_type "Output Data Type"; addr_width "Address width"; data_width "Data Width"; reg_prim_output "Register Primitive Output"; reg_core_output "Register Core Output"; data_bin_pt "Data Binary Point"; init_vals "Initial 32-bit values (simulation only)"; sample_rate "Sample rate"
      mask init:
      | shared_bram_mask;
      mask TypeOptions arith_type: Unsigned | Signed  (2's comp)
      mask TypeOptions data_width: 8 | 16 | 32 | 64 | 128
      mask TypeOptions optimization: Minimum_Area | Low_Power
  coeff_real : Subsystem  Tag=xps:bram  AncestorBlock=xps_library/Shared BRAM  mask{arith_type=Unsigned, addr_width=10, data_width=32, reg_prim_output=on, reg_core_output=on, optimization=Minimum_Area, data_bin_pt=0, init_vals=[0:2^10-1], sample_rate=1}
      mask prompts: arith_type "Output Data Type"; addr_width "Address width"; data_width "Data Width"; reg_prim_output "Register Primitive Output"; reg_core_output "Register Core Output"; data_bin_pt "Data Binary Point"; init_vals "Initial 32-bit values (simulation only)"; sample_rate "Sample rate"
      mask init:
      | shared_bram_mask;
      mask TypeOptions arith_type: Unsigned | Signed  (2's comp)
      mask TypeOptions data_width: 8 | 16 | 32 | 64 | 128
      mask TypeOptions optimization: Minimum_Area | Low_Power
  pipeline1 : Subsystem  AncestorBlock=casper_library_delays/pipeline  mask(pipeline){latency=1}
      mask help:
      | An explicitly laid-out delay line to avoid mapping to SRL16s
      | for use in pipelining to help achieve timing closure.
      mask init:
      | pipeline_init(gcb,'latency',latency);
      settings: AttributesFormatString=Latency = %<latency>
      mask Display:
      | port_label('input', 1, 'd');
      | port_label('output', 1, 'q');
      | disp(['Z^-', num2str(latency)]);
  pipeline2 : Subsystem  AncestorBlock=casper_library_delays/pipeline  mask(pipeline){latency=1}
      mask help:
      | An explicitly laid-out delay line to avoid mapping to SRL16s
      | for use in pipelining to help achieve timing closure.
      mask init:
      | pipeline_init(gcb,'latency',latency);
      settings: AttributesFormatString=Latency = %<latency>
      mask Display:
      | port_label('input', 1, 'd');
      | port_label('output', 1, 'q');
      | disp(['Z^-', num2str(latency)]);
  ri_to_c : casper_library_misc/ri_to_c
  dout : Outport
  sync_out : Outport  Port=2
  wires:
  Counter/1 -> coeff_imag/1(addr), coeff_real/1(addr)
  sync_in/1 -> Counter/1, amp_scale/1(sync)
  Constant/1 -> coeff_real/3(we)
  Constant1/1 -> coeff_real/2(data_in)
  Constant3/1 -> coeff_imag/2(data_in)
  Constant2/1 -> coeff_imag/3(we)
  din/1 -> Delay1/1
  amp_scale/2(Out) -> dout/1
  ri_to_c/1 -> amp_scale/3(scale)
  amp_scale/1(synchOut) -> sync_out/1
  Delay1/1 -> Delay2/1
  Delay2/1 -> amp_scale/2(din)
  Slice/1 -> Concat/1
  Slice3/1 -> Concat/2
  Concat/1 -> Reinterpret/1
  pipeline2/1(q) -> Slice3/1, Slice/1
  Slice1/1 -> Concat1/1
  Slice2/1 -> Concat1/2
  Concat1/1 -> Reinterpret1/1
  pipeline1/1(q) -> Slice1/1, Slice2/1
  coeff_real/1(data_out) -> pipeline2/1(d)
  coeff_imag/1(data_out) -> pipeline1/1(d)
  Reinterpret/1 -> ri_to_c/1
  Reinterpret1/1 -> ri_to_c/2

== system rx_20140505/amp_EQ2 ==
  sync_in : Inport
  din : Inport  Port=2
  Concat : xbsIndex_r4/Concat  num_inputs=2  dbl_ovrd=off  block_type=concat
  Concat1 : xbsIndex_r4/Concat  num_inputs=2  dbl_ovrd=off  block_type=concat
  Constant : xbsIndex_r4/Constant  const=0  gui_display_data_type=Fixed-point  arith_type=Boolean  n_bits=16  bin_pt=14  preci_type=Single  exp_width=8  frac_width=24  explicit_period=on  period=1  equ=P=C  opselect=C  inp2=PCIN>>17  opr=+  inp1=P  carry=CIN  dbl_ovrd=off  block_type=constant
      settings: block_version=11.4
  Constant1 : xbsIndex_r4/Constant  const=0  gui_display_data_type=Fixed-point  arith_type=Unsigned  n_bits=32  bin_pt=0  preci_type=Single  exp_width=8  frac_width=24  explicit_period=on  period=1  equ=P=C  opselect=C  inp2=PCIN>>17  opr=+  inp1=P  carry=CIN  dbl_ovrd=off  block_type=constant
      settings: block_version=11.4
  Constant2 : xbsIndex_r4/Constant  const=0  gui_display_data_type=Fixed-point  arith_type=Boolean  n_bits=16  bin_pt=14  preci_type=Single  exp_width=8  frac_width=24  explicit_period=on  period=1  equ=P=C  opselect=C  inp2=PCIN>>17  opr=+  inp1=P  carry=CIN  dbl_ovrd=off  block_type=constant
      settings: block_version=11.4
  Constant3 : xbsIndex_r4/Constant  const=0  gui_display_data_type=Fixed-point  arith_type=Unsigned  n_bits=32  bin_pt=0  preci_type=Single  exp_width=8  frac_width=24  explicit_period=on  period=1  equ=P=C  opselect=C  inp2=PCIN>>17  opr=+  inp1=P  carry=CIN  dbl_ovrd=off  block_type=constant
      settings: block_version=11.4
  Counter : xbsIndex_r4/Counter  cnt_type=Free Running  cnt_to=Inf  operation=Up  start_count=0  cnt_by_val=1  arith_type=Unsigned  n_bits=N  bin_pt=0  load_pin=off  rst=on  en=off  explicit_period=on  period=1  dbl_ovrd=off  use_behavioral_HDL=off  implementation=Fabric  block_type=counter
      settings: block_version=11.4
  Delay1 : xbsIndex_r4/Delay  rst=off  infoeditControl=Selection of Reset will increase slice count due to use of real FFs and instead of SRLs  en=off  latency=1  dbl_ovrd=off  reg_retiming=off  block_type=delay
      settings: block_version=11.4
  Delay2 : xbsIndex_r4/Delay  rst=off  infoeditControl=Selection of Reset will increase slice count due to use of real FFs and instead of SRLs  en=off  latency=1  dbl_ovrd=off  reg_retiming=off  block_type=delay
      settings: block_version=11.4
  Reinterpret : xbsIndex_r4/Reinterpret  force_arith_type=on  arith_type="Signed  (2's comp)"  force_bin_pt=off  bin_pt=0  block_type=reinterpret
      settings: infoedit="Changes signal type without altering the binary representation.   You can changed the signal between signed and unsigned, and relocate the binary point.<br><br>Hardware notes: In hardware this block costs nothing.<br><br>Example:  Suppose the input is 6 bits wide, signed, with 2 fractional bits, and the output is forced to unsigned with 0 fractional bits.  Then an input of -2.0 (1110.00 in binary 2's complement) becomes an output of 56 (111000 in binary)."
  Reinterpret1 : xbsIndex_r4/Reinterpret  force_arith_type=on  arith_type="Signed  (2's comp)"  force_bin_pt=off  bin_pt=0  block_type=reinterpret
      settings: infoedit="Changes signal type without altering the binary representation.   You can changed the signal between signed and unsigned, and relocate the binary point.<br><br>Hardware notes: In hardware this block costs nothing.<br><br>Example:  Suppose the input is 6 bits wide, signed, with 2 fractional bits, and the output is forced to unsigned with 0 fractional bits.  Then an input of -2.0 (1110.00 in binary 2's complement) becomes an output of 56 (111000 in binary)."
  Slice : xbsIndex_r4/Slice  nbits=1  boolean_output=off  mode=Upper Bit Location + Width  bit1=0  base1=MSB of Input  bit0=0  base0=LSB of Input  dbl_ovrd=off  block_type=slice
  Slice1 : xbsIndex_r4/Slice  nbits=1  boolean_output=off  mode=Upper Bit Location + Width  bit1=0  base1=MSB of Input  bit0=0  base0=LSB of Input  dbl_ovrd=off  block_type=slice
  Slice2 : xbsIndex_r4/Slice  nbits=12  boolean_output=off  mode=Lower Bit Location + Width  bit1=0  base1=MSB of Input  bit0=0  base0=LSB of Input  dbl_ovrd=off  block_type=slice
  Slice3 : xbsIndex_r4/Slice  nbits=12  boolean_output=off  mode=Lower Bit Location + Width  bit1=0  base1=MSB of Input  bit0=0  base0=LSB of Input  dbl_ovrd=off  block_type=slice
  amp_scale : Subsystem  mask{add_latency=2, mult_latency=3, bit_width=18, scale_bit_width=13}
      mask prompts: bit_width "bit_width_data"; scale_bit_width "bit_width_Scaling"
      mask init:
      | add_latency=2;
      | mult_latency=3;
  coeff_imag : Subsystem  Tag=xps:bram  AncestorBlock=xps_library/Shared BRAM  mask{arith_type=Unsigned, addr_width=10, data_width=32, reg_prim_output=on, reg_core_output=on, optimization=Minimum_Area, data_bin_pt=0, init_vals=[0:2^10-1], sample_rate=1}
      mask prompts: arith_type "Output Data Type"; addr_width "Address width"; data_width "Data Width"; reg_prim_output "Register Primitive Output"; reg_core_output "Register Core Output"; data_bin_pt "Data Binary Point"; init_vals "Initial 32-bit values (simulation only)"; sample_rate "Sample rate"
      mask init:
      | shared_bram_mask;
      mask TypeOptions arith_type: Unsigned | Signed  (2's comp)
      mask TypeOptions data_width: 8 | 16 | 32 | 64 | 128
      mask TypeOptions optimization: Minimum_Area | Low_Power
  coeff_real : Subsystem  Tag=xps:bram  AncestorBlock=xps_library/Shared BRAM  mask{arith_type=Unsigned, addr_width=10, data_width=32, reg_prim_output=on, reg_core_output=on, optimization=Minimum_Area, data_bin_pt=0, init_vals=[0:2^10-1], sample_rate=1}
      mask prompts: arith_type "Output Data Type"; addr_width "Address width"; data_width "Data Width"; reg_prim_output "Register Primitive Output"; reg_core_output "Register Core Output"; data_bin_pt "Data Binary Point"; init_vals "Initial 32-bit values (simulation only)"; sample_rate "Sample rate"
      mask init:
      | shared_bram_mask;
      mask TypeOptions arith_type: Unsigned | Signed  (2's comp)
      mask TypeOptions data_width: 8 | 16 | 32 | 64 | 128
      mask TypeOptions optimization: Minimum_Area | Low_Power
  pipeline1 : Subsystem  AncestorBlock=casper_library_delays/pipeline  mask(pipeline){latency=1}
      mask help:
      | An explicitly laid-out delay line to avoid mapping to SRL16s
      | for use in pipelining to help achieve timing closure.
      mask init:
      | pipeline_init(gcb,'latency',latency);
      settings: AttributesFormatString=Latency = %<latency>
      mask Display:
      | port_label('input', 1, 'd');
      | port_label('output', 1, 'q');
      | disp(['Z^-', num2str(latency)]);
  pipeline2 : Subsystem  AncestorBlock=casper_library_delays/pipeline  mask(pipeline){latency=1}
      mask help:
      | An explicitly laid-out delay line to avoid mapping to SRL16s
      | for use in pipelining to help achieve timing closure.
      mask init:
      | pipeline_init(gcb,'latency',latency);
      settings: AttributesFormatString=Latency = %<latency>
      mask Display:
      | port_label('input', 1, 'd');
      | port_label('output', 1, 'q');
      | disp(['Z^-', num2str(latency)]);
  ri_to_c : casper_library_misc/ri_to_c
  dout : Outport
  sync_out : Outport  Port=2
  wires:
  Counter/1 -> coeff_imag/1(addr), coeff_real/1(addr)
  sync_in/1 -> Counter/1, amp_scale/1(sync)
  Constant/1 -> coeff_real/3(we)
  Constant1/1 -> coeff_real/2(data_in)
  Constant3/1 -> coeff_imag/2(data_in)
  Constant2/1 -> coeff_imag/3(we)
  din/1 -> Delay1/1
  amp_scale/2(Out) -> dout/1
  ri_to_c/1 -> amp_scale/3(scale)
  amp_scale/1(synchOut) -> sync_out/1
  Delay1/1 -> Delay2/1
  Delay2/1 -> amp_scale/2(din)
  Slice/1 -> Concat/1
  Slice3/1 -> Concat/2
  Concat/1 -> Reinterpret/1
  pipeline2/1(q) -> Slice3/1, Slice/1
  Slice1/1 -> Concat1/1
  Slice2/1 -> Concat1/2
  Concat1/1 -> Reinterpret1/1
  pipeline1/1(q) -> Slice1/1, Slice2/1
  coeff_real/1(data_out) -> pipeline2/1(d)
  coeff_imag/1(data_out) -> pipeline1/1(d)
  Reinterpret/1 -> ri_to_c/1
  Reinterpret1/1 -> ri_to_c/2
